simulink model "heli_q8_4_2_output"  (Simulink 8.3)
settings: Solver=ode1  StartTime=0.0  StopTime=inf  FixedStep=0.002  RelTol=1e-3
PostLoadFcn:
  | qc_set_target_type(getConfigSet(bdroot, 'QUARC Default Target Configuration'));
undefined symbols (not defined in the file): A_0, B_0, C_0, HIL, Joystick_gain_x, Joystick_gain_y, K, L, P, qc_get_step_size
libraries: simulink_extras x6, quarc_library x4
settings Model: Creator=Rchan  LastModifiedBy=hongyuz  SimulationMode=external  ExtModeTrigDuration=500000
settings SolverCC: PositivePriorityOrder=on
settings DataIOCC: MaxDataPoints=1000000
settings OptimizationCC: ExpressionDepthLimit=2147483647  InitFltsAndDblsToZero=on
settings DebuggingCC: SaveWithParameterizedLinksMsg=none  MultiTaskDSMMsg=warning  MultiTaskCondExecSysMsg=none  FcnCallInpInsideContextMsg=UseLocalSettings
settings RTWCC: SystemTargetFile=quarc_win64.tlc  TemplateMakefile=quarc_default_tmf  Description=QUARC Win64 Target  ProcessScript=quarc_win64_make_rtw_hook
settings STFCustomTargetCC: TargetPreCompLibLocation=C:\PROGRA~3\QUARC\lib\2014a\win64\release  ConcurrentExecutionCompliant=on  GeneratePreprocessorConditionals=Disable all  CPPClassGenCompliant=on  SystemTargetFile=quarc_win64.tlc
settings GRTTargetCC: TargetPreCompLibLocation=C:\PROGRA~3\QUARC\lib\2014a\win64\release  ParMdlRefBuildCompliant=off  CompOptLevelCompliant=off  MatFileLogging=off  ExtMode=on  ExtModeMexFile=quarc_comm

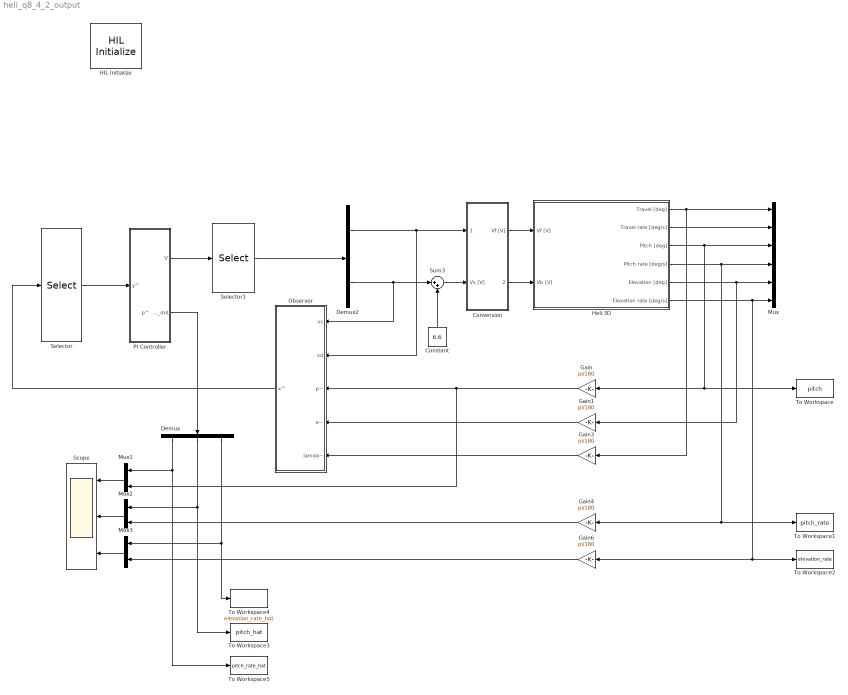
== system heli_q8_4_2_output ==
  Constant : Constant  Value=6.6
  Conversion : Subsystem
  Demux : Demux  Outputs=3
  Demux2 : Demux  Outputs=2
  Gain{,1,3..4,6} (5 alike) : Gain  Gain=pi/180
  HIL Initialize : quarc_library/Data Acquisition/Generic/Configuration/HIL Initialize  Priority=-99  object_name=HIL-1  board_type=q8_usb  board_number=0  board_options=update_rate=normal;decimation=1  exclusive=off  active=off  hardware_clocks=[0:2]  clock_modes=[]  initial_clock_frequencies=[]  set_clock_params_at_start=off  set_clock_params_at_switch_in=off  set_clock_frequencies_at_start=off  set_clock_frequencies_at_switch_in=off  analog_input_channels=[0:7]  analog_input_maximums=10  analog_input_minimums=-10  set_analog_input_params_at_start=on  set_analog_input_params_at_switch_in=off  analog_output_channels=[0:7]  analog_output_maximums=10  analog_output_minimums=-10  initial_analog_outputs=[0]  final_analog_outputs=[0]  watchdog_analog_outputs=0  set_analog_output_params_at_start=on  set_analog_output_params_at_switch_in=off  set_analog_outputs_at_start=on  set_analog_outputs_at_switch_in=off  set_analog_outputs_at_terminate=on  set_analog_outputs_at_switch_out=off  set_analog_outputs_on_watchdog=off  digital_input_channels=[]  digital_output_channels=[]  digital_output_configuration=[]  initial_digital_outputs=[1]  final_digital_outputs=[1]  watchdog_digital_outputs=[1]  set_digital_output_params_at_start=off  set_digital_output_params_at_switch_in=off  set_digital_outputs_at_start=on  set_digital_outputs_at_switch_in=off  set_digital_outputs_at_terminate=on  set_digital_outputs_at_switch_out=off  set_digital_outputs_on_watchdog=off  encoder_channels=[0:7]  quadrature=[4]  encoder_filter_frequency=[]  initial_encoder_counts=[0]  set_encoder_params_at_start=on  set_encoder_params_at_switch_in=off  set_encoder_counts_at_start=on  set_encoder_counts_at_switch_in=off  pwm_channels=[0:7]  pwm_modes=0  pwm_frequency=99.532799999999995e6/4095  pwm_configuration=[0]  pwm_alignment=[0]  pwm_polarity=[1]  pwm_leading_deadband=[0]  pwm_trailing_deadband=[0]  initial_pwm_outputs=[0]  final_pwm_outputs=[0]  watchdog_pwm_outputs=[0]  set_pwm_params_at_start=on  set_pwm_params_at_switch_in=off  set_pwm_outputs_at_start=on  set_pwm_outputs_at_switch_in=off  set_pwm_outputs_at_terminate=on  set_pwm_outputs_at_switch_out=off  set_pwm_outputs_on_watchdog=off  other_output_channels=[]  initial_other_outputs=[]  final_other_outputs=[]  watchdog_other_outputs=[]  set_other_outputs_at_start=off  set_other_outputs_at_switch_in=off  set_other_outputs_at_terminate=off  set_other_outputs_at_switch_out=off  set_other_outputs_on_watchdog=off
  Heli 3D : Subsystem
  Mux : Mux  Inputs=6
  Mux1 : Mux  Inputs=2
  Mux2 : Mux  Inputs=2
  Mux3 : Mux  Inputs=2
  Observor : Subsystem
  PI Controller : Subsystem
  Scope : Scope  NumInputPorts=3
      settings: Priority=3  YMin=-5~-5~-5  YMax=5~5~5
  Selector : Selector  InputPortWidth=6  Indices=[1 2 4]
  Selector1 : Selector  InputPortWidth=2  Indices=[2 1]
  Sum3 : Sum  Inputs=|++
  To Workspace : ToWorkspace  VariableName=pitch  SaveFormat=Structure With Time  SampleTime=-1
  To Workspace1 : ToWorkspace  VariableName=pitch_rate  SaveFormat=Structure With Time  SampleTime=-1
  To Workspace2 : ToWorkspace  VariableName=elevation_rate  SaveFormat=Structure With Time  SampleTime=-1
  To Workspace3 : ToWorkspace  VariableName=pitch_hat  SaveFormat=Structure With Time  SampleTime=-1
  To Workspace4 : ToWorkspace  VariableName=elevation_rate_hat  SaveFormat=Structure With Time  SampleTime=-1
  To Workspace5 : ToWorkspace  VariableName=pitch_rate_hat  SaveFormat=Structure With Time  SampleTime=-1
  wires:
  Heli 3D/1(Travel [deg]) -> Mux/1, Gain3/1
  Heli 3D/2(Travel rate [deg/s]) -> Mux/2
  Heli 3D/4(Pitch rate [deg/s]) -> Mux/4, Gain4/1, To Workspace1/1
  Heli 3D/5(Elevation [deg]) -> Mux/5, Gain1/1
  Heli 3D/6(Elevation rate [deg/s]) -> Gain6/1, To Workspace2/1, Mux/6
  Conversion/1(Vf [V]) -> Heli 3D/1(Vf [V])
  Conversion/2(Vb [V]) -> Heli 3D/2(Vb [V])
  Heli 3D/3(Pitch [deg]) -> Gain/1, To Workspace/1, Mux/3
  Mux1/1 -> Scope/1
  Mux2/1 -> Scope/2
  Gain4/1 -> Mux2/2
  Gain6/1 -> Mux3/2
  Sum3/1 -> Conversion/2(Vs [V])
  Constant/1 -> Sum3/2
  Observor/1(x^) -> Selector/1
  Gain1/1 -> Observor/4(e~)
  Gain3/1 -> Observor/5(lamda~)
  Mux3/1 -> Scope/3
  Gain/1 -> Mux1/2, Observor/3(p~)
  Selector/1 -> PI Controller/1(y^)
  Selector1/1 -> Demux2/1
  Demux2/1 -> Observor/2(vd), Conversion/1(Vd [V])
  Demux2/2 -> Observor/1(vs), Sum3/1
  PI Controller/1(V) -> Selector1/1
  PI Controller/2(p^  p^_dot  e^_dot) -> Demux/1
  Demux/1 -> To Workspace5/1, Mux1/1
  Demux/2 -> Mux2/1, To Workspace3/1
  Demux/3 -> Mux3/1, To Workspace4/1

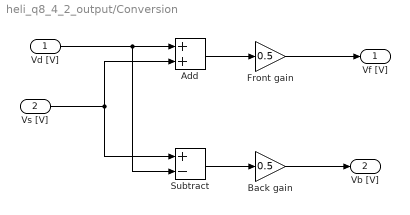
== system heli_q8_4_2_output/Conversion ==
  Vd [V] : Inport
  Vs [V] : Inport  Port=2
  Add : Sum
  Back gain : Gain  Gain=0.5
  Front gain : Gain  Gain=0.5
  Subtract : Sum  Inputs=+-
  Vf [V] : Outport
  Vb [V] : Outport  Port=2
  wires:
  Vd [V]/1 -> Subtract/2, Add/1
  Vs [V]/1 -> Subtract/1, Add/2
  Subtract/1 -> Back gain/1
  Back gain/1 -> Vb [V]/1
  Add/1 -> Front gain/1
  Front gain/1 -> Vf [V]/1

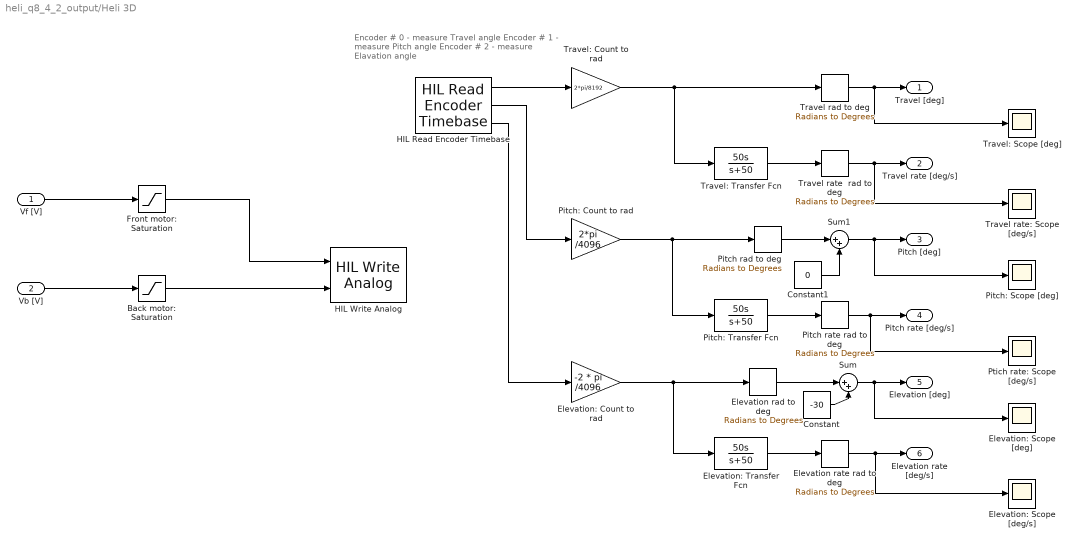
== system heli_q8_4_2_output/Heli 3D ==
  note: Encoder # 0 - measure Travel angle
      | Encoder # 1 - measure Pitch angle
      | Encoder # 2 - measure Elavation angle
  Vf [V] : Inport
  Vb [V] : Inport  Port=2
  Back motor: Saturation : Saturate  UpperLimit=5  LowerLimit=-5
  Constant : Constant  Value=-30
  Constant1 : Constant  Value=0
  Elevation rad to deg : simulink_extras/Transformations/Radians to Degrees
  Elevation rate rad to deg : simulink_extras/Transformations/Radians to Degrees
  Elevation: Count to rad : Gain  Gain=-2 * pi /4096
  Elevation: Scope [deg/s] : Scope
      settings: YMin=-15  YMax=15  SaveName=ScopeData13
  Elevation: Scope [deg] : Scope
      settings: YMin=-2.1  YMax=-0.6  SaveName=ScopeData12
  Elevation: Transfer Fcn : TransferFcn  Numerator=[50 0]  Denominator=[1 50]
  Front motor: Saturation : Saturate  UpperLimit=5  LowerLimit=-5
  HIL Read Encoder Timebase : quarc_library/Data Acquisition/Generic/Timebases/HIL Read Encoder Timebase  object_name=HIL-1  clock=0  channels=[0:2]  samples_in_buffer=max(ceil(1/qc_get_step_size), 1)  active=on  vector_output=off  data_type_mode=Inherit via back propagation  data_type=double
  HIL Write Analog : quarc_library/Data Acquisition/Generic/Immediate I//O/HIL Write Analog  object_name=HIL-1  channels=[0:1]  sample_time=-1  active=off  vector_input=off
  Pitch rad to deg : simulink_extras/Transformations/Radians to Degrees
  Pitch rate rad to deg : simulink_extras/Transformations/Radians to Degrees
  Pitch: Count to rad : Gain  Gain=2*pi /4096
  Pitch: Scope [deg] : Scope
      settings: YMin=-15  YMax=15  SaveName=ScopeData10
  Pitch: Transfer Fcn : TransferFcn  Numerator=[50 0]  Denominator=[1 50]
  Ptich rate: Scope [deg/s] : Scope
      settings: YMin=-15  YMax=15  SaveName=ScopeData11
  Sum : Sum  Inputs=|++
  Sum1 : Sum  Inputs=|++
  Travel rad to deg : simulink_extras/Transformations/Radians to Degrees
  Travel rate  rad to deg : simulink_extras/Transformations/Radians to Degrees
  Travel rate: Scope [deg/s] : Scope
      settings: YMin=-15  YMax=15  SaveName=ScopeData9
  Travel: Count to rad : Gain  Gain=2*pi/8192
  Travel: Scope [deg] : Scope
      settings: TimeRange=30  YMin=0  YMax=350  SaveName=ScopeData8
  Travel: Transfer Fcn : TransferFcn  Numerator=[50 0]  Denominator=[1 50]
  Travel [deg] : Outport
  Travel rate [deg/s] : Outport  Port=2
  Pitch [deg] : Outport  Port=3
  Pitch rate [deg/s] : Outport  Port=4
  Elevation [deg] : Outport  Port=5
  Elevation rate [deg/s] : Outport  Port=6
  wires:
  HIL Read Encoder Timebase/1 -> Travel: Count to rad/1
  HIL Read Encoder Timebase/2 -> Pitch: Count to rad/1
  HIL Read Encoder Timebase/3 -> Elevation: Count to rad/1
  Travel: Count to rad/1 -> Travel: Transfer Fcn/1, Travel rad to deg/1
  Travel: Transfer Fcn/1 -> Travel rate  rad to deg/1
  Pitch: Count to rad/1 -> Pitch: Transfer Fcn/1, Pitch rad to deg/1
  Pitch: Transfer Fcn/1 -> Pitch rate rad to deg/1
  Elevation: Count to rad/1 -> Elevation: Transfer Fcn/1, Elevation rad to deg/1
  Elevation: Transfer Fcn/1 -> Elevation rate rad to deg/1
  Travel rad to deg/1 -> Travel: Scope [deg]/1, Travel [deg]/1
  Travel rate  rad to deg/1 -> Travel rate: Scope [deg/s]/1, Travel rate [deg/s]/1
  Pitch rate rad to deg/1 -> Pitch rate [deg/s]/1, Ptich rate: Scope [deg/s]/1
  Elevation rate rad to deg/1 -> Elevation: Scope [deg/s]/1, Elevation rate [deg/s]/1
  Vf [V]/1 -> Front motor: Saturation/1
  Vb [V]/1 -> Back motor: Saturation/1
  Front motor: Saturation/1 -> HIL Write Analog/1
  Back motor: Saturation/1 -> HIL Write Analog/2
  Sum/1 -> Elevation: Scope [deg]/1, Elevation [deg]/1
  Elevation rad to deg/1 -> Sum/1
  Constant/1 -> Sum/2
  Pitch rad to deg/1 -> Sum1/1
  Constant1/1 -> Sum1/2
  Sum1/1 -> Pitch: Scope [deg]/1, Pitch [deg]/1

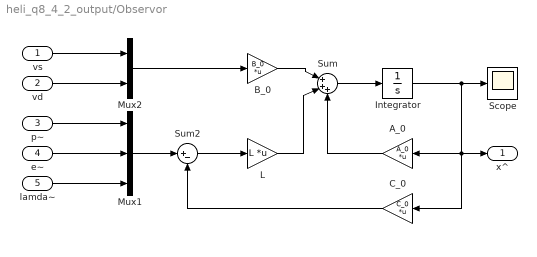
== system heli_q8_4_2_output/Observor ==
  vs : Inport
  vd : Inport  Port=2
  p~ : Inport  Port=3
  e~ : Inport  Port=4
  lamda~ : Inport  Port=5
  A_0 : Gain  Gain=A_0  Multiplication=Matrix(K*u)
  B_0 : Gain  Gain=B_0  Multiplication=Matrix(K*u)
  C_0 : Gain  Gain=C_0  Multiplication=Matrix(K*u)
  Integrator : Integrator
  L : Gain  Gain=L  Multiplication=Matrix(K*u)
  Mux1 : Mux  Inputs=3
  Mux2 : Mux  Inputs=2
  Scope : Scope
  Sum : Sum  Inputs=|+++
  Sum2 : Sum  Inputs=|+-
  x^ : Outport
  wires:
  p~/1 -> Mux1/1
  e~/1 -> Mux1/2
  lamda~/1 -> Mux1/3
  Mux1/1 -> Sum2/1
  C_0/1 -> Sum2/2
  Sum2/1 -> L/1
  L/1 -> Sum/2
  Sum/1 -> Integrator/1
  Integrator/1 -> x^/1, C_0/1, A_0/1, Scope/1
  A_0/1 -> Sum/3
  vs/1 -> Mux2/1
  vd/1 -> Mux2/2
  Mux2/1 -> B_0/1
  B_0/1 -> Sum/1

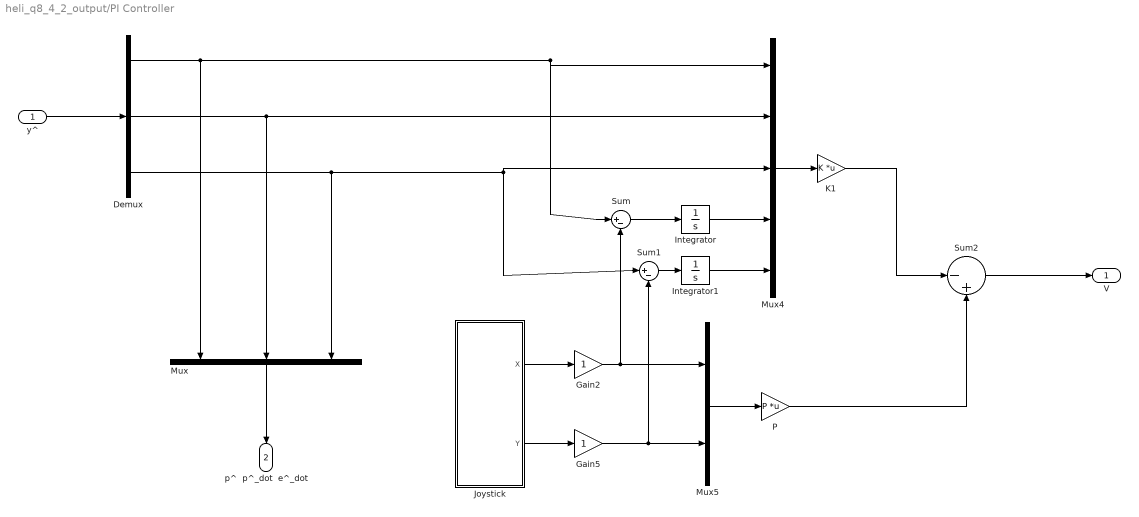
== system heli_q8_4_2_output/PI Controller ==
  y^ : Inport
  Demux : Demux  Outputs=3
  Gain2 : Gain
  Gain5 : Gain
  Integrator : Integrator
  Integrator1 : Integrator
  Joystick : Subsystem
  K1 : Gain  Gain=K  Multiplication=Matrix(K*u)
  Mux : Mux  Inputs=3
  Mux4 : Mux  Inputs=5
  Mux5 : Mux  Inputs=2
  P : Gain  Gain=P  Multiplication=Matrix(K*u)
  Sum : Sum  Inputs=|+-
  Sum1 : Sum  Inputs=|+-
  Sum2 : Sum  Inputs=|-+
  V : Outport
  p^  p^_dot  e^_dot : Outport  Port=2
  wires:
  K1/1 -> Sum2/1
  Joystick/1(X) -> Gain2/1
  Joystick/2(Y) -> Gain5/1
  Demux/3 -> Mux/3, Mux4/3, Sum1/1
  Integrator/1 -> Mux4/4
  Integrator1/1 -> Mux4/5
  Sum1/1 -> Integrator1/1
  Sum/1 -> Integrator/1
  Gain2/1 -> Mux5/1, Sum/2
  Gain5/1 -> Sum1/2, Mux5/2
  Mux5/1 -> P/1
  Mux4/1 -> K1/1
  P/1 -> Sum2/2
  Demux/1 -> Mux/1, Sum/1, Mux4/1
  Demux/2 -> Mux/2, Mux4/2
  y^/1 -> Demux/1
  Sum2/1 -> V/1
  Mux/1 -> p^  p^_dot  e^_dot/1

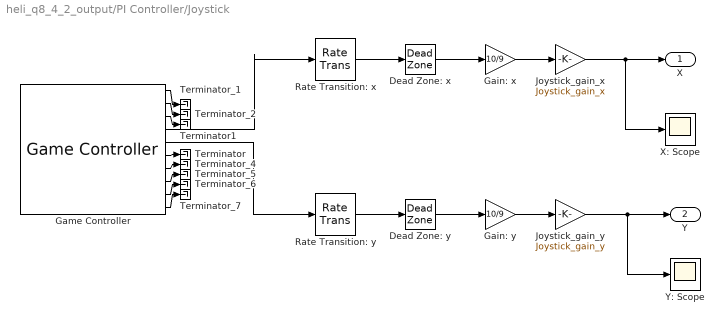
== system heli_q8_4_2_output/PI Controller/Joystick ==
  Dead Zone: x : DeadZone  LowerValue=-0.1  UpperValue=0.1  SaturateOnIntegerOverflow=on
  Dead Zone: y : DeadZone  LowerValue=-0.1  UpperValue=0.1  SaturateOnIntegerOverflow=on
  Gain: x : Gain  Gain=10/9
  Gain: y : Gain  Gain=10/9
  Game Controller : quarc_library/Devices/Peripherals/Target/Game Controller  controller=1  buffer_size=12  deadzone=[]  saturation=[]  sample_time=max(qc_get_step_size, 0.01)  auto_center=off  enabled=on
  Joystick_gain_x : Gain  Gain=Joystick_gain_x
  Joystick_gain_y : Gain  Gain=Joystick_gain_y
  Rate Transition: x : RateTransition
  Rate Transition: y : RateTransition
  Terminator : Terminator
  Terminator1 : Terminator
  Terminator_{1..2,4..7} (6 alike) : Terminator
  X: Scope : Scope
      settings: YMin=-1  YMax=1  SaveName=ScopeData7
  Y: Scope : Scope
      settings: YMin=-10  YMax=10  SaveName=ScopeData5
  X : Outport
  Y : Outport  Port=2
  wires:
  Rate Transition: y/1 -> Dead Zone: y/1
  Rate Transition: x/1 -> Dead Zone: x/1
  Game Controller/5 -> Rate Transition: y/1
  Game Controller/4 -> Rate Transition: x/1
  Game Controller/1 -> Terminator_1/1
  Game Controller/2 -> Terminator_2/1
  Game Controller/7 -> Terminator_4/1
  Game Controller/8 -> Terminator_5/1
  Game Controller/9 -> Terminator_6/1
  Game Controller/10 -> Terminator_7/1
  Game Controller/3 -> Terminator1/1
  Game Controller/6 -> Terminator/1
  Dead Zone: x/1 -> Gain: x/1
  Dead Zone: y/1 -> Gain: y/1
  Gain: x/1 -> Joystick_gain_x/1
  Gain: y/1 -> Joystick_gain_y/1
  Joystick_gain_x/1 -> X/1, X: Scope/1
  Joystick_gain_y/1 -> Y: Scope/1, Y/1
